simulink model "dx_hand_model"  (R2017b)
settings: Solver=ode3  StartTime=0.0  StopTime=inf  FixedStep=0.01  RelTol=1e-3  EnableMultiTasking=on
InitFcn:
  | cutFreq = 0.1; % T
  | sampleTime = 0.01;
  | filt = tf(1,[cutFreq 1]);
  | filt = c2d(filt,sampleTime);
  | 
  | cutFreq2 = 1;
  | filt2 = tf(1,[cutFreq2 1]);
  | filt2 = c2d(filt2,sampleTime);
  | 
  | cutFreq3 = 0.3;
  | filt3 = tf(1,[cutFreq3 1]);
  | filt3 = c2d(filt3,sampleTime);
  | 
  | update_param = 2;
  | 
  | ampliFactor = 1.60;
  | ampliFactorMiddle = 2.00;
  | ampliFactorDistal = 1;
  | 
  | % Set Hand Address
  | % RightHandAddress = '10.100.39.144';
  | RightHandAddress = '10.24.4.91';
  | Verosim = '10.100.39.22'
  | LeftHandAddress = '10.100.39.22'
  | 
  | max_force = 24; % Newton
model workspace (MAT data in the model file):
  SL_ROS_VariableLengthArrays_MaxSizes : struct (value not decoded)
libraries: robotlib x136, simulink_extras x27, simulink x16, etargetslib x2, dspnetwork x2
(part 15 of 19)

== matlab function dx_hand_model/Thumb/Direct Kinematics/F transformation new ==
  data: B output; C output; q_A input; F output; q_B input; F_1 output; q_C input; D output; E output; q_E input; q_J input; J output; I output
function [B,C,F,F_1, D, E, J, I]  = fcn(q_A, q_B, q_C, q_E, q_J)
T_B =[ - (4967757600021511*sin(q_A))/40564819207303340847894502572032 - (2^(1/2)*cos(q_A))/2,                                  2^(1/2)/2 - (24678615572571482867467662723121*cos(q_A))/3291009114642412084309938365114701009965471731267159726697218048 + (4967757600021511*2^(1/2)*sin(q_A))/162259276829213363391578010288128,                          (4967757600021511*cos(q_A))/40564819207303340847894502572032 + (4967757600021511*2^(1/2))/162259276829213363391578010288128 - (2^(1/2)*sin(q_A))/2,                                        (33*2^(1/2))/4;...
               (7025470172532439*cos(q_A))/81129638414606681695789005144064 - sin(q_A), - (4967757600021511*cos(q_A))/81129638414606681695789005144064 - (34900832843322459977667745295329*sin(q_A))/6582018229284824168619876730229402019930943462534319453394436096 - 7025470172532437/81129638414606681695789005144064, cos(q_A) + (7025470172532439*sin(q_A))/81129638414606681695789005144064 - 34900832843322450042152545252307/6582018229284824168619876730229402019930943462534319453394436096, -231840515693570421/162259276829213363391578010288128;...
                                                                  (2^(1/2)*cos(q_A))/2,                                                                                                                                                 2^(1/2)/2 - (4967757600021511*2^(1/2)*sin(q_A))/162259276829213363391578010288128,                                                                                         (4967757600021511*2^(1/2))/162259276829213363391578010288128 + (2^(1/2)*sin(q_A))/2,                                        (33*2^(1/2))/4;...
                                                                                     0,                                                                                                                                                                                                                                 0,                                                                                                                                                                           0,                                                     1]; 

T_C = [                    sin(q_B + pi/2)*(2^(1/2)/2 - (24678615572571482867467662723121*cos(q_A))/3291009114642412084309938365114701009965471731267159726697218048 + (4967757600021511*2^(1/2)*sin(q_A))/162259276829213363391578010288128) - cos(q_B + pi/2)*((4967757600021511*sin(q_A))/40564819207303340847894502572032 + (2^(1/2)*cos(q_A))/2),                      cos(q_B + pi/2)*(2^(1/2)/2 - (24678615572571482867467662723121*cos(q_A))/3291009114642412084309938365114701009965471731267159726697218048 + (4967757600021511*2^(1/2)*sin(q_A))/162259276829213363391578010288128) + sin(q_B + pi/2)*((4967757600021511*sin(q_A))/40564819207303340847894502572032 + (2^(1/2)*cos(q_A))/2),                          (4967757600021511*cos(q_A))/40564819207303340847894502572032 + (4967757600021511*2^(1/2))/162259276829213363391578010288128 - (2^(1/2)*sin(q_A))/2,                                                          (33*2^(1/2))/4 - 30*cos(q_B + pi/2)*((4967757600021511*sin(q_A))/40564819207303340847894502572032 + (2^(1/2)*cos(q_A))/2) + 30*sin(q_B + pi/2)*(2^(1/2)/2 - (24678615572571482867467662723121*cos(q_A))/3291009114642412084309938365114701009965471731267159726697218048 + (4967757600021511*2^(1/2)*sin(q_A))/162259276829213363391578010288128);...
 cos(q_B + pi/2)*((7025470172532439*cos(q_A))/81129638414606681695789005144064 - sin(q_A)) - sin(q_B + pi/2)*((4967757600021511*cos(q_A))/81129638414606681695789005144064 + (34900832843322459977667745295329*sin(q_A))/6582018229284824168619876730229402019930943462534319453394436096 + 7025470172532437/81129638414606681695789005144064), - cos(q_B + pi/2)*((4967757600021511*cos(q_A))/81129638414606681695789005144064 + (34900832843322459977667745295329*sin(q_A))/6582018229284824168619876730229402019930943462534319453394436096 + 7025470172532437/81129638414606681695789005144064) - sin(q_B + pi/2)*((7025470172532439*cos(q_A))/81129638414606681695789005144064 - sin(q_A)), cos(q_A) + (7025470172532439*sin(q_A))/81129638414606681695789005144064 - 34900832843322450042152545252307/6582018229284824168619876730229402019930943462534319453394436096, 30*cos(q_B + pi/2)*((7025470172532439*cos(q_A))/81129638414606681695789005144064 - sin(q_A)) - 30*sin(q_B + pi/2)*((4967757600021511*cos(q_A))/81129638414606681695789005144064 + (34900832843322459977667745295329*sin(q_A))/6582018229284824168619876730229402019930943462534319453394436096 + 7025470172532437/81129638414606681695789005144064) - 231840515693570421/162259276829213363391578010288128;...
                                                                                                                                                                                                    sin(q_B + pi/2)*(2^(1/2)/2 - (4967757600021511*2^(1/2)*sin(q_A))/162259276829213363391578010288128) + (2^(1/2)*cos(q_A)*cos(q_B + pi/2))/2,                                                                                                                                                                                                      cos(q_B + pi/2)*(2^(1/2)/2 - (4967757600021511*2^(1/2)*sin(q_A))/162259276829213363391578010288128) - (2^(1/2)*cos(q_A)*sin(q_B + pi/2))/2,                                                                                         (4967757600021511*2^(1/2))/162259276829213363391578010288128 + (2^(1/2)*sin(q_A))/2,                                                                                                                                                                                                                                              30*sin(q_B + pi/2)*(2^(1/2)/2 - (4967757600021511*2^(1/2)*sin(q_A))/162259276829213363391578010288128) + (33*2^(1/2))/4 + 15*2^(1/2)*cos(q_A)*cos(q_B + pi/2);...
                                                                                                                                                                                                                                                                                                                                 0,                                                                                                                                                                                                                                                                                                                                               0,                                                                                                                                                                           0,                                                                                                                                                                                                                                                                                                                                                                                                          1];
                                                                                                                                                                                                                                                                                                                                             
A_3 = [ cos(q_C - 2305491947385741/1125899906842624), -sin(q_C - 2305491947385741/1125899906842624), 0, 4561^(1/2)*cos(q_C - 2305491947385741/1125899906842624); ...
 sin(q_C - 2305491947385741/1125899906842624),  cos(q_C - 2305491947385741/1125899906842624), 0, 4561^(1/2)*sin(q_C - 2305491947385741/1125899906842624); ...
                                            0,                                             0, 1,                                                       0; ...
                                            0,                                             0, 0,                                                       1];
 
A_4 = [ cos(q_C - pi/2), -(4967757600021511*sin(q_C - pi/2))/81129638414606681695789005144064,                                  -sin(q_C - pi/2), 60*cos(q_C - pi/2); ...
 sin(q_C - pi/2),  (4967757600021511*cos(q_C - pi/2))/81129638414606681695789005144064,                                   cos(q_C - pi/2), 60*sin(q_C - pi/2); ...
0,                                                                   -1, 4967757600021511/81129638414606681695789005144064,                  0; ...
               0,                                                                    0,                                                 0,                  1];
 
A_D = [ cos(q_C - pi/2), -(4967757600021511*sin(q_C - pi/2))/81129638414606681695789005144064,                                  -sin(q_C - pi/2), 85*cos(q_C - pi/2); ...
 sin(q_C - pi/2),  (4967757600021511*cos(q_C - pi/2))/81129638414606681695789005144064,                                   cos(q_C - pi/2), 85*sin(q_C - pi/2); ...
               0,                                                                   -1, 4967757600021511/81129638414606681695789005144064,                  0; ...
               0,                                                                    0,                                                 0,                  1];
 
C_E = [0.0000    0.0000    1.0000   33.5857; ...
   -1.0000    0.0000    0.0000  -91.0000; ...
         0   -1.0000    0.0000    0.0000; ...
         0         0         0    1.0000];

E_J = [ cos(q_E), -(4967757600021511*sin(q_E))/81129638414606681695789005144064,                                          sin(q_E), 100*cos(q_E); ...
 sin(q_E),  (4967757600021511*cos(q_E))/81129638414606681695789005144064,                                         -cos(q_E), 100*sin(q_E); ...
        0,                                                             1, 4967757600021511/81129638414606681695789005144064,            0; ...
        0,                                                             0,                                                 0,            1];

J_I = [ 0, 0, 0,  80*sin(q_J); ...
 0, 0, 0, -80*cos(q_J); ...
 0, 0, 0,            0; ...
 0, 0, 0,            1];

T_F = T_C*A_3;
T_F_1 = T_C*A_4;
T_D = T_C*A_D;
T_E = T_C*C_E;
T_J = T_E*E_J;
T_I = T_J*J_I;

B = T_B*[ 0, 0, 0, 1]';
C = T_C*[ 0, 0, 0, 1]';
F = T_F*[ 0, 0, 0, 1]';
F_1 = T_F_1*[ 0, 0, 0, 1]';
D = T_D*[0, 0, 0, 1]';                                                                                                                                                                                                                                                                                                                                                                                                                                                                                                                                                                                                                                                                                                                                                                                         
E = T_E*[0, 0, 0, 1]';
J = T_J*[0,0,0,1]';
I = T_I*[0,0,0,1]';
end

== matlab function dx_hand_model/Thumb/Metacarphal Phalanx/MATLAB Function1 ==
  data: u input; d output
function d = fcn(u)

d = sqrt(u(1)^2+u(2)^2+u(3)^2);

== matlab function dx_hand_model/Thumb/Direct Kinematics/get H/MATLAB Function5 ==
  data: u input; d output
function d = fcn(u)

d = sqrt(u(1)^2+u(2)^2+u(3)^2);

== matlab function dx_hand_model/Thumb/Direct Kinematics/get H/MATLAB Function6 ==
  data: u input; d output
function d = fcn(u)

d = sqrt(u(1)^2+u(2)^2+u(3)^2);

== matlab function dx_hand_model/Thumb/Direct Kinematics/get H/MATLAB Function7 ==
  data: u input; d output
function d = fcn(u)

d = sqrt(u(1)^2+u(2)^2+u(3)^2);

== matlab function dx_hand_model/Thumb/Direct Kinematics/get H/MATLAB Function8 ==
  data: u input; d output
function d = fcn(u)

d = sqrt(u(1)^2+u(2)^2+u(3)^2);

== matlab function dx_hand_model/Thumb/Direct Kinematics/get H/MATLAB Function9 ==
  data: a input; xH output; b input; yH output; zH output
function [xH,yH,zH] = fcn(a,b)
if a(2) > b(2)
    xH = a(1);
    yH = a(2);
    zH = a(3);
else
    xH = b(1);
    yH = b(2);
    zH = b(3);
end

== matlab function dx_hand_model/Thumb/Direct Kinematics/get H/MATLAB Function10 ==
  data: u input; d output
function d = fcn(u)

d = sqrt(u(1)^2+u(2)^2+u(3)^2);

== matlab function dx_hand_model/Thumb/Direct Kinematics/Get G/MATLAB Function ==
  data: xI input; yI input; zI input; xH input; yH input; zH input; xD input; yD input; zD input; xG2_sol output; yG2_sol output; zG2_sol output
function [xG2_sol,yG2_sol,zG2_sol] = findG2_optimized(xI,yI,zI,xH,yH, zH, xD,yD, zD )
%function [xG2_sol,yG2_sol,zG2_sol] = findG2_optimized(xD,xH,xI,yD,yH,yI,zD,zH,zI)
%FINDG2_OPTIMIZED
%    [XG2_SOL,YG2_SOL,ZG2_SOL] = FINDG2_OPTIMIZED(XD,XH,XI,YD,YH,YI,ZD,ZH,ZI)

%    This function was generated by the Symbolic Math Toolbox version 8.0.
%    16-Feb-2018 10:54:09

t2 = xD.^2;
t3 = xH.^2;
t4 = zD.^2;
t5 = zH.^2;
t6 = yD.^2;
t7 = yI.^2;
t8 = xI.^2;
t9 = yH.^2;
t10 = zI.^2;
t11 = t4.^2;
t12 = t5.^2;
t13 = t2.*t9.*5.329e3;
t14 = t3.*t6.*5.329e3;
t15 = t2.*t7.*5.329e3;
t16 = t6.*t8.*5.329e3;
t17 = t3.*t7.*5.329e3;
t18 = t8.*t9.*5.329e3;
t19 = t2.*t5.*5.329e3;
t20 = t3.*t4.*5.329e3;
t21 = t2.*t10.*5.329e3;
t22 = t4.*t8.*5.329e3;
t23 = t3.*t10.*5.329e3;
t24 = t5.*t8.*5.329e3;
t25 = t5.*t6.*5.329e3;
t26 = t4.*t9.*5.329e3;
t27 = t6.*t10.*5.329e3;
t28 = t4.*t7.*5.329e3;
t29 = t9.*t10.*5.329e3;
t30 = t5.*t7.*5.329e3;
t31 = xD.*xH.*yD.*yI.*1.0658e4;
t32 = xD.*xI.*yD.*yH.*1.0658e4;
t33 = xD.*xH.*yH.*yI.*1.0658e4;
t34 = xH.*xI.*yD.*yH.*1.0658e4;
t35 = xD.*xI.*yH.*yI.*1.0658e4;
t36 = xH.*xI.*yD.*yI.*1.0658e4;
t37 = xD.*xH.*zD.*zI.*1.0658e4;
t38 = xD.*xI.*zD.*zH.*1.0658e4;
t39 = xD.*xH.*zH.*zI.*1.0658e4;
t40 = xH.*xI.*zD.*zH.*1.0658e4;
t41 = xD.*xI.*zH.*zI.*1.0658e4;
t42 = xH.*xI.*zD.*zI.*1.0658e4;
t43 = yD.*yH.*zD.*zI.*1.0658e4;
t44 = yD.*yI.*zD.*zH.*1.0658e4;
t45 = yD.*yH.*zH.*zI.*1.0658e4;
t46 = yH.*yI.*zD.*zH.*1.0658e4;
t47 = yD.*yI.*zH.*zI.*1.0658e4;
t48 = yH.*yI.*zD.*zI.*1.0658e4;
t74 = t7.*xD.*xH.*1.0658e4;
t75 = t9.*xD.*xI.*1.0658e4;
t76 = t6.*xH.*xI.*1.0658e4;
t77 = t10.*xD.*xH.*1.0658e4;
t78 = t5.*xD.*xI.*1.0658e4;
t79 = t4.*xH.*xI.*1.0658e4;
t80 = t2.*yH.*yI.*1.0658e4;
t81 = t3.*yD.*yI.*1.0658e4;
t82 = t8.*yD.*yH.*1.0658e4;
t83 = t10.*yD.*yH.*1.0658e4;
t84 = t5.*yD.*yI.*1.0658e4;
t85 = t4.*yH.*yI.*1.0658e4;
t86 = t2.*zH.*zI.*1.0658e4;
t87 = t3.*zD.*zI.*1.0658e4;
t88 = t8.*zD.*zH.*1.0658e4;
t89 = t6.*zH.*zI.*1.0658e4;
t90 = t9.*zD.*zI.*1.0658e4;
t91 = t7.*zD.*zH.*1.0658e4;
t92 = xD.*xH.*yD.*yH.*1.0658e4;
t93 = xD.*xI.*yD.*yI.*1.0658e4;
t94 = xH.*xI.*yH.*yI.*1.0658e4;
t95 = xD.*xH.*zD.*zH.*1.0658e4;
t96 = xD.*xI.*zD.*zI.*1.0658e4;
t97 = xH.*xI.*zH.*zI.*1.0658e4;
t98 = yD.*yH.*zD.*zH.*1.0658e4;
t99 = yD.*yI.*zD.*zI.*1.0658e4;
t100 = yH.*yI.*zH.*zI.*1.0658e4;
t49 = t13+t14+t15+t16+t17+t18+t19+t20+t21+t22+t23+t24+t25+t26+t27+t28+t29+t30+t31+t32+t33+t34+t35+t36+t37+t38+t39+t40+t41+t42+t43+t44+t45+t46+t47+t48-t74-t75-t76-t77-t78-t79-t80-t81-t82-t83-t84-t85-t86-t87-t88-t89-t90-t91-t92-t93-t94-t95-t96-t97-t98-t99-t100;
t203 = t2.*t5.*zH.*7.592e3;
t204 = t3.*t4.*zD.*3.066e3;
t205 = t4.*t8.*zD.*3.066e3;
t206 = t5.*t8.*zH.*7.592e3;
t207 = t5.*t6.*zH.*7.592e3;
t208 = t4.*t9.*zD.*3.066e3;
t209 = t4.*t7.*zD.*3.066e3;
t210 = t5.*t7.*zH.*7.592e3;
t211 = t5.*xD.*xI.*zH.*1.5184e4;
t212 = t4.*xH.*xI.*zD.*6.132e3;
t213 = t5.*yD.*yI.*zH.*1.5184e4;
t214 = t4.*yH.*yI.*zD.*6.132e3;
t215 = t2.*t9.*zD.*3.066e3;
t216 = t3.*t6.*zD.*3.066e3;
t217 = t2.*t7.*zD.*3.066e3;
t218 = t6.*t8.*zD.*3.066e3;
t219 = t2.*t9.*zH.*7.592e3;
t220 = t3.*t6.*zH.*7.592e3;
t221 = t2.*t7.*zH.*7.592e3;
t222 = t3.*t7.*zD.*3.066e3;
t223 = t6.*t8.*zH.*7.592e3;
t224 = t8.*t9.*zD.*3.066e3;
t225 = t3.*t7.*zH.*7.592e3;
t226 = t8.*t9.*zH.*7.592e3;
t227 = t2.*t5.*zD.*3.066e3;
t228 = t2.*t10.*zD.*3.066e3;
t229 = t3.*t4.*zH.*7.592e3;
t230 = t2.*t10.*zH.*7.592e3;
t231 = t2.*t5.*zI.*1.5184e4;
t232 = t3.*t10.*zD.*3.066e3;
t233 = t3.*t4.*zI.*6.132e3;
t234 = t5.*t8.*zD.*1.2118e4;
t235 = t4.*t8.*zH.*1.46e3;
t236 = t3.*t10.*zH.*7.592e3;
t237 = t5.*t6.*zD.*3.066e3;
t238 = t6.*t10.*zD.*3.066e3;
t239 = t4.*t9.*zH.*7.592e3;
t240 = t6.*t10.*zH.*7.592e3;
t241 = t5.*t6.*zI.*1.5184e4;
t242 = t9.*t10.*zD.*3.066e3;
t243 = t4.*t9.*zI.*6.132e3;
t244 = t5.*t7.*zD.*1.2118e4;
t245 = t4.*t7.*zH.*1.46e3;
t246 = t9.*t10.*zH.*7.592e3;
t247 = t7.*xD.*xH.*zD.*6.132e3;
t248 = t9.*xD.*xI.*zD.*6.132e3;
t249 = t6.*xH.*xI.*zD.*6.132e3;
t250 = t7.*xD.*xH.*zH.*1.5184e4;
t251 = t9.*xD.*xI.*zH.*1.5184e4;
t252 = t6.*xH.*xI.*zH.*1.5184e4;
t253 = t5.*xD.*xH.*zD.*1.5184e4;
t254 = t4.*xD.*xH.*zH.*6.132e3;
t255 = t10.*xD.*xH.*zD.*6.132e3;
t256 = t4.*xD.*xH.*zI.*6.132e3;
t257 = t5.*xD.*xI.*zD.*9.052e3;
t258 = t4.*xD.*xI.*zH.*6.132e3;
t259 = t2.*yH.*yI.*zD.*6.132e3;
t260 = t3.*yD.*yI.*zD.*6.132e3;
t261 = t8.*yD.*yH.*zD.*6.132e3;
t262 = t4.*xD.*xI.*zI.*6.132e3;
t263 = t10.*xD.*xH.*zH.*1.5184e4;
t264 = t5.*xD.*xH.*zI.*1.5184e4;
t265 = t5.*xH.*xI.*zD.*1.5184e4;
t266 = t4.*xH.*xI.*zH.*9.052e3;
t267 = t2.*yH.*yI.*zH.*1.5184e4;
t268 = t3.*yD.*yI.*zH.*1.5184e4;
t269 = t8.*yD.*yH.*zH.*1.5184e4;
t270 = t5.*xD.*xI.*zI.*1.5184e4;
t271 = t4.*xH.*xI.*zI.*6.132e3;
t272 = t5.*xH.*xI.*zI.*1.5184e4;
t273 = t5.*yD.*yH.*zD.*1.5184e4;
t274 = t4.*yD.*yH.*zH.*6.132e3;
t275 = t10.*yD.*yH.*zD.*6.132e3;
t276 = t4.*yD.*yH.*zI.*6.132e3;
t277 = t5.*yD.*yI.*zD.*9.052e3;
t278 = t4.*yD.*yI.*zH.*6.132e3;
t279 = t2.*zD.*zH.*zI.*6.132e3;
t280 = t4.*yD.*yI.*zI.*6.132e3;
t281 = t10.*yD.*yH.*zH.*1.5184e4;
t282 = t5.*yD.*yH.*zI.*1.5184e4;
t283 = t5.*yH.*yI.*zD.*1.5184e4;
t284 = t4.*yH.*yI.*zH.*9.052e3;
t285 = t3.*zD.*zH.*zI.*1.5184e4;
t286 = t5.*yD.*yI.*zI.*1.5184e4;
t287 = t4.*yH.*yI.*zI.*6.132e3;
t288 = t5.*yH.*yI.*zI.*1.5184e4;
t289 = t6.*zD.*zH.*zI.*6.132e3;
t290 = t9.*zD.*zH.*zI.*1.5184e4;
t291 = xD.*xH.*yD.*yH.*zD.*6.132e3;
t292 = xD.*xH.*yD.*yI.*zD.*6.132e3;
t293 = xD.*xI.*yD.*yH.*zD.*6.132e3;
t294 = xD.*xI.*yD.*yI.*zD.*6.132e3;
t295 = xD.*xH.*yD.*yH.*zH.*1.5184e4;
t296 = xD.*xH.*yD.*yI.*zH.*1.5184e4;
t297 = xD.*xH.*yH.*yI.*zD.*6.132e3;
t298 = xD.*xI.*yD.*yH.*zH.*1.5184e4;
t299 = xH.*xI.*yD.*yH.*zD.*6.132e3;
t300 = xD.*xI.*yD.*yI.*zH.*1.5184e4;
t301 = xD.*xI.*yH.*yI.*zD.*6.132e3;
t302 = xH.*xI.*yD.*yI.*zD.*6.132e3;
t303 = xD.*xH.*yH.*yI.*zH.*1.5184e4;
t304 = xH.*xI.*yD.*yH.*zH.*1.5184e4;
t305 = xD.*xI.*yH.*yI.*zH.*1.5184e4;
t306 = xH.*xI.*yD.*yI.*zH.*1.5184e4;
t307 = xH.*xI.*yH.*yI.*zD.*6.132e3;
t308 = xH.*xI.*yH.*yI.*zH.*1.5184e4;
t309 = xD.*xH.*zD.*zH.*zI.*2.1316e4;
t310 = xD.*xI.*zD.*zH.*zI.*9.052e3;
t311 = xH.*xI.*zD.*zH.*zI.*9.052e3;
t312 = yD.*yH.*zD.*zH.*zI.*2.1316e4;
t313 = yD.*yI.*zD.*zH.*zI.*9.052e3;
t314 = yH.*yI.*zD.*zH.*zI.*9.052e3;
t50 = t203+t204+t205+t206+t207+t208+t209+t210-t211-t212-t213-t214+t215+t216+t217+t218+t219+t220+t221+t222+t223+t224+t225+t226+t227+t228+t229+t230-t231+t232-t233-t234+t235+t236+t237+t238+t239+t240-t241+t242-t243-t244+t245+t246-t247-t248-t249-t250-t251-t252-t253-t254-t255+t256+t257+t258-t259-t260-t261-t262-t263+t264+t265-t266-t267-t268-t269+t270+t271-t272-t273-t274-t275+t276+t277+t278-t279-t280-t281+t282+t283-t284-t285+t286+t287-t288-t289-t290-t291+t292+t293-t294-t295+t296+t297+t298+t299-t300+t301+t302+t303+t304+t305+t306-t307-t308+t309-t310+t311+t312-t313+t314;
t51 = xD.*yH;
t52 = xI.*yD;
t53 = xH.*yI;
t56 = xH.*yD;
t57 = xD.*yI;
t58 = xI.*yH;
t54 = t51+t52+t53-t56-t57-t58;
t55 = 1.0./t54;
t59 = t3.*yD.*5.2e1;
t60 = t2.*yI.*2.1e1;
t61 = t5.*yD.*5.2e1;
t62 = t4.*yI.*2.1e1;
t63 = xD.*xH.*yD.*2.1e1;
t64 = xD.*xH.*yI.*3.1e1;
t65 = xD.*xI.*yH.*2.1e1;
t66 = xH.*xI.*yH.*5.2e1;
t67 = yD.*zD.*zH.*2.1e1;
t68 = yH.*zD.*zI.*2.1e1;
t69 = yI.*zD.*zH.*3.1e1;
t70 = yH.*zH.*zI.*5.2e1;
t71 = t59+t60+t61+t62+t63+t64+t65+t66+t67+t68+t69+t70-t2.*yH.*2.1e1-t4.*yH.*2.1e1-t3.*yI.*5.2e1-t5.*yI.*5.2e1-xD.*xI.*yD.*2.1e1-xD.*xH.*yH.*5.2e1-xH.*xI.*yD.*5.2e1-yD.*zD.*zI.*2.1e1-yH.*zD.*zH.*5.2e1-yD.*zH.*zI.*5.2e1;
t72 = zD.*(2.1e1./7.3e1);
t73 = zH.*(5.2e1./7.3e1);
t101 = 1.0./t49;
t102 = t2.*t12.*2.704e3;
t103 = t3.*t11.*4.41e2;
t104 = t8.*t11.*4.41e2;
t105 = t8.*t12.*2.704e3;
t106 = t6.*t12.*2.704e3;
t107 = t9.*t11.*4.41e2;
t108 = t7.*t11.*4.41e2;
t109 = t7.*t12.*2.704e3;
t110 = t7.*xD.*xH.*1.0913792e7;
t111 = t9.*xD.*xI.*1.0913792e7;
t112 = t6.*xH.*xI.*1.0913792e7;
t113 = t2.*yH.*yI.*1.0913792e7;
t114 = t3.*yD.*yI.*1.0913792e7;
t115 = t8.*yD.*yH.*1.0913792e7;
t116 = t2.*t5.*zD.*zH.*2.184e3;
t117 = t3.*t4.*zD.*zH.*2.184e3;
t118 = t4.*t8.*zD.*zH.*1.302e3;
t119 = t5.*t6.*zD.*zH.*2.184e3;
t120 = t4.*t9.*zD.*zH.*2.184e3;
t121 = t4.*t7.*zD.*zH.*1.302e3;
t122 = t2.*t4.*t9.*4.41e2;
t123 = t3.*t4.*t6.*4.41e2;
t124 = t2.*t4.*t7.*4.41e2;
t125 = t4.*t6.*t8.*4.41e2;
t126 = t2.*t5.*t9.*2.704e3;
t127 = t3.*t5.*t6.*2.704e3;
t128 = t2.*t5.*t7.*2.704e3;
t129 = t3.*t4.*t7.*4.41e2;
t130 = t5.*t6.*t8.*2.704e3;
t131 = t4.*t8.*t9.*4.41e2;
t132 = t3.*t5.*t7.*2.704e3;
t133 = t5.*t8.*t9.*2.704e3;
t134 = t2.*t4.*t5.*4.41e2;
t135 = t2.*t4.*t10.*4.41e2;
t136 = t3.*t4.*t5.*2.704e3;
t137 = t2.*t5.*t10.*2.704e3;
t138 = t3.*t4.*t10.*4.41e2;
t139 = t3.*t5.*t10.*2.704e3;
t140 = t4.*t5.*t6.*4.41e2;
t141 = t4.*t6.*t10.*4.41e2;
t142 = t4.*t5.*t9.*2.704e3;
t143 = t5.*t6.*t10.*2.704e3;
t144 = t4.*t9.*t10.*4.41e2;
t145 = t5.*t9.*t10.*2.704e3;
t146 = t4.*t5.*xD.*xI.*3.486e3;
t147 = t2.*t9.*zD.*zH.*2.184e3;
t148 = t3.*t6.*zD.*zH.*2.184e3;
t149 = t2.*t7.*zD.*zH.*2.184e3;
t150 = t6.*t8.*zD.*zH.*2.184e3;
t151 = t3.*t7.*zD.*zH.*2.184e3;
t152 = t8.*t9.*zD.*zH.*2.184e3;
t153 = t4.*t5.*yD.*yI.*3.486e3;
t154 = t2.*t10.*zD.*zH.*2.184e3;
t155 = t3.*t10.*zD.*zH.*2.184e3;
t156 = t6.*t10.*zD.*zH.*2.184e3;
t157 = t9.*t10.*zD.*zH.*2.184e3;
t158 = xD.*xH.*yD.*yH.*1.0913792e7;
t159 = xD.*xI.*yD.*yI.*1.0913792e7;
t160 = xH.*xI.*yH.*yI.*1.0913792e7;
t161 = t4.*xD.*xH.*zD.*zI.*8.82e2;
t162 = t5.*xD.*xI.*zD.*zH.*1.04e3;
t163 = t4.*xD.*xI.*zD.*zH.*8.82e2;
t164 = t5.*xD.*xH.*zH.*zI.*5.408e3;
t165 = t5.*xH.*xI.*zD.*zH.*5.408e3;
t166 = t5.*xD.*xI.*zH.*zI.*5.408e3;
t167 = t4.*xH.*xI.*zD.*zI.*8.82e2;
t168 = t4.*yD.*yH.*zD.*zI.*8.82e2;
t169 = t5.*yD.*yI.*zD.*zH.*1.04e3;
t170 = t4.*yD.*yI.*zD.*zH.*8.82e2;
t171 = t5.*yD.*yH.*zH.*zI.*5.408e3;
t172 = t5.*yH.*yI.*zD.*zH.*5.408e3;
t173 = t5.*yD.*yI.*zH.*zI.*5.408e3;
t174 = t4.*yH.*yI.*zD.*zI.*8.82e2;
t175 = t4.*xD.*xH.*yD.*yI.*8.82e2;
t176 = t4.*xD.*xI.*yD.*yH.*8.82e2;
t177 = t5.*xD.*xH.*yD.*yI.*5.408e3;
t178 = t4.*xD.*xH.*yH.*yI.*8.82e2;
t179 = t5.*xD.*xI.*yD.*yH.*5.408e3;
t180 = t4.*xH.*xI.*yD.*yH.*8.82e2;
t181 = t4.*xD.*xI.*yH.*yI.*8.82e2;
t182 = t4.*xH.*xI.*yD.*yI.*8.82e2;
t183 = t5.*xD.*xH.*yH.*yI.*5.408e3;
t184 = t5.*xH.*xI.*yD.*yH.*5.408e3;
t185 = t5.*xD.*xI.*yH.*yI.*5.408e3;
t186 = t5.*xH.*xI.*yD.*yI.*5.408e3;
t187 = t5.*xD.*xH.*zD.*zI.*9.776e3;
t188 = t4.*xD.*xH.*zH.*zI.*5.25e3;
t189 = t5.*xH.*xI.*zD.*zI.*1.04e3;
t190 = t4.*xH.*xI.*zH.*zI.*3.486e3;
t191 = t5.*yD.*yH.*zD.*zI.*9.776e3;
t192 = t4.*yD.*yH.*zH.*zI.*5.25e3;
t193 = t5.*yH.*yI.*zD.*zI.*1.04e3;
t194 = t4.*yH.*yI.*zH.*zI.*3.486e3;
t195 = xD.*xH.*yD.*yI.*zD.*zH.*4.368e3;
t196 = xD.*xI.*yD.*yH.*zD.*zH.*4.368e3;
t197 = xD.*xH.*yH.*yI.*zD.*zH.*4.368e3;
t198 = xH.*xI.*yD.*yH.*zD.*zH.*4.368e3;
t199 = xD.*xI.*yH.*yI.*zD.*zH.*4.368e3;
t200 = xH.*xI.*yD.*yI.*zD.*zH.*4.368e3;
t323 = t2.*t9.*5.456896e6;
t324 = t3.*t6.*5.456896e6;
t325 = t2.*t7.*5.456896e6;
t326 = t6.*t8.*5.456896e6;
t327 = t3.*t7.*5.456896e6;
t328 = t8.*t9.*5.456896e6;
t329 = t12.*xD.*xI.*5.408e3;
t330 = t11.*xH.*xI.*8.82e2;
t331 = t12.*yD.*yI.*5.408e3;
t332 = t11.*yH.*yI.*8.82e2;
t333 = t2.*t5.*zH.*zI.*5.408e3;
t334 = t3.*t4.*zD.*zI.*8.82e2;
t335 = t5.*t8.*zD.*zH.*3.224e3;
t336 = t5.*t6.*zH.*zI.*5.408e3;
t337 = t4.*t9.*zD.*zI.*8.82e2;
t338 = t5.*t7.*zD.*zH.*3.224e3;
t339 = t4.*t5.*t8.*1.223e3;
t340 = t4.*t5.*t7.*1.223e3;
t341 = t4.*t7.*xD.*xH.*8.82e2;
t342 = t4.*t9.*xD.*xI.*8.82e2;
t343 = t4.*t6.*xH.*xI.*8.82e2;
t344 = t5.*t7.*xD.*xH.*5.408e3;
t345 = t5.*t9.*xD.*xI.*5.408e3;
t346 = t5.*t6.*xH.*xI.*5.408e3;
t347 = t4.*t5.*xD.*xH.*4.368e3;
t348 = t4.*t10.*xD.*xH.*8.82e2;
t349 = t2.*t4.*yH.*yI.*8.82e2;
t350 = t3.*t4.*yD.*yI.*8.82e2;
t351 = t4.*t8.*yD.*yH.*8.82e2;
t352 = t5.*t10.*xD.*xH.*5.408e3;
t353 = t4.*t5.*xH.*xI.*1.04e3;
t354 = t2.*t5.*yH.*yI.*5.408e3;
t355 = t3.*t5.*yD.*yI.*5.408e3;
t356 = t5.*t8.*yD.*yH.*5.408e3;
t357 = t4.*t5.*yD.*yH.*4.368e3;
t358 = t4.*t10.*yD.*yH.*8.82e2;
t359 = t2.*t5.*zD.*zI.*4.368e3;
t360 = t2.*t4.*zH.*zI.*8.82e2;
t361 = t5.*t10.*yD.*yH.*5.408e3;
t362 = t4.*t5.*yH.*yI.*1.04e3;
t363 = t3.*t5.*zD.*zI.*5.408e3;
t364 = t3.*t4.*zH.*zI.*4.368e3;
t365 = t5.*t6.*zD.*zI.*4.368e3;
t366 = t4.*t6.*zH.*zI.*8.82e2;
t367 = t5.*t9.*zD.*zI.*5.408e3;
t368 = t4.*t9.*zH.*zI.*4.368e3;
t369 = xD.*xH.*yD.*yI.*1.0913792e7;
t370 = xD.*xI.*yD.*yH.*1.0913792e7;
t371 = xD.*xH.*yH.*yI.*1.0913792e7;
t372 = xH.*xI.*yD.*yH.*1.0913792e7;
t373 = xD.*xI.*yH.*yI.*1.0913792e7;
t374 = xH.*xI.*yD.*yI.*1.0913792e7;
t375 = t5.*xD.*xH.*zD.*zH.*5.408e3;
t376 = t4.*xD.*xH.*zD.*zH.*8.82e2;
t377 = t4.*xD.*xI.*zD.*zI.*8.82e2;
t378 = t4.*xH.*xI.*zD.*zH.*3.486e3;
t379 = t5.*xH.*xI.*zH.*zI.*5.408e3;
t380 = t5.*yD.*yH.*zD.*zH.*5.408e3;
t381 = t4.*yD.*yH.*zD.*zH.*8.82e2;
t382 = t4.*yD.*yI.*zD.*zI.*8.82e2;
t383 = t4.*yH.*yI.*zD.*zH.*3.486e3;
t384 = t5.*yH.*yI.*zH.*zI.*5.408e3;
t385 = t4.*xD.*xH.*yD.*yH.*8.82e2;
t386 = t4.*xD.*xI.*yD.*yI.*8.82e2;
t387 = t5.*xD.*xH.*yD.*yH.*5.408e3;
t388 = t5.*xD.*xI.*yD.*yI.*5.408e3;
t389 = t4.*xH.*xI.*yH.*yI.*8.82e2;
t390 = t5.*xH.*xI.*yH.*yI.*5.408e3;
t391 = t7.*xD.*xH.*zD.*zH.*4.368e3;
t392 = t9.*xD.*xI.*zD.*zH.*4.368e3;
t393 = t6.*xH.*xI.*zD.*zH.*4.368e3;
t394 = t10.*xD.*xH.*zD.*zH.*4.368e3;
t395 = t2.*yH.*yI.*zD.*zH.*4.368e3;
t396 = t3.*yD.*yI.*zD.*zH.*4.368e3;
t397 = t8.*yD.*yH.*zD.*zH.*4.368e3;
t398 = t5.*xD.*xI.*zD.*zI.*1.04e3;
t399 = t4.*xD.*xI.*zH.*zI.*3.486e3;
t400 = t10.*yD.*yH.*zD.*zH.*4.368e3;
t401 = t5.*yD.*yI.*zD.*zI.*1.04e3;
t402 = t4.*yD.*yI.*zH.*zI.*3.486e3;
t403 = xD.*xH.*yD.*yH.*zD.*zH.*4.368e3;
t404 = xD.*xI.*yD.*yI.*zD.*zH.*4.368e3;
t405 = xH.*xI.*yH.*yI.*zD.*zH.*4.368e3;
t201 = t102+t103+t104+t105+t106+t107+t108+t109+t110+t111+t112+t113+t114+t115+t116+t117+t118+t119+t120+t121+t122+t123+t124+t125+t126+t127+t128+t129+t130+t131+t132+t133+t134+t135+t136+t137+t138+t139+t140+t141+t142+t143+t144+t145+t146+t147+t148+t149+t150+t151+t152+t153+t154+t155+t156+t157+t158+t159+t160+t161+t162+t163+t164+t165+t166+t167+t168+t169+t170+t171+t172+t173+t174+t175+t176+t177+t178+t179+t180+t181+t182+t183+t184+t185+t186+t187+t188+t189+t190+t191+t192+t193+t194+t195+t196+t197+t198+t199+t200-t323-t324-t325-t326-t327-t328-t329-t330-t331-t332-t333-t334-t335-t336-t337-t338-t339-t340-t341-t342-t343-t344-t345-t346-t347-t348-t349-t350-t351-t352-t353-t354-t355-t356-t357-t358-t359-t360-t361-t362-t363-t364-t365-t366-t367-t368-t369-t370-t371-t372-t373-t374-t375-t376-t377-t378-t379-t380-t381-t382-t383-t384-t385-t386-t387-t388-t389-t390-t391-t392-t393-t394-t395-t396-t397-t398-t399-t400-t401-t402-t403-t404-t405;
t202 = 1.0./t49.^2;
t315 = t50.^2;
t316 = t202.*t315.*(1.0./4.0);
t406 = t101.*t201;
t317 = t316-t406;
t318 = sqrt(complex(t317));
t319 = yD.*zH;
t320 = yI.*zD;
t321 = yH.*zI;
t322 = t319+t320+t321-yH.*zD-yD.*zI-yI.*zH;
t407 = t72+t73+t318;
t408 = t9.*xD.*5.2e1;
t409 = t6.*xI.*2.1e1;
t410 = t5.*xD.*5.2e1;
t411 = t4.*xI.*2.1e1;
t412 = xD.*yD.*yH.*2.1e1;
t413 = xH.*yD.*yI.*2.1e1;
t414 = xI.*yD.*yH.*3.1e1;
t415 = xH.*yH.*yI.*5.2e1;
t416 = xD.*zD.*zH.*2.1e1;
t417 = xH.*zD.*zI.*2.1e1;
t418 = xI.*zD.*zH.*3.1e1;
t419 = xH.*zH.*zI.*5.2e1;
t420 = t408+t409+t410+t411+t412+t413+t414+t415+t416+t417+t418+t419-t4.*xH.*2.1e1-t6.*xH.*2.1e1-t5.*xI.*5.2e1-t9.*xI.*5.2e1-xD.*yD.*yI.*2.1e1-xH.*yD.*yH.*5.2e1-xD.*yH.*yI.*5.2e1-xD.*zD.*zI.*2.1e1-xH.*zD.*zH.*5.2e1-xD.*zH.*zI.*5.2e1;
t421 = t55.*t420.*(1.0./7.3e1);
t422 = t72+t73-t318;
xG2_sol = [t55.*t71.*(-1.0./7.3e1)+t55.*t322.*t407;t55.*t71.*(-1.0./7.3e1)+t55.*t322.*t422];
if nargout > 1
    t423 = xD.*zH;
    t424 = xI.*zD;
    t425 = xH.*zI;
    t426 = t423+t424+t425-xH.*zD-xD.*zI-xI.*zH;
    yG2_sol = [t421-t55.*t407.*t426;t421-t55.*t422.*t426];
end
if nargout > 2
    zG2_sol = [t407;t422];
end

== matlab function dx_hand_model/Thumb/Direct Kinematics/Get G/MATLAB Function2 ==
  data: x output; u input; y output; z output
function [x,y,z] = split(u)

x = u(1);
y = u(2);
z = u(3);

== matlab function dx_hand_model/Thumb/Direct Kinematics/Get G/MATLAB Function1 ==
  data: x output; u input; y output; z output
function [x,y,z] = split(u)

x = u(1);
y = u(2);
z = u(3);

== matlab function dx_hand_model/Thumb/Direct Kinematics/Get G/MATLAB Function4 ==
  data: u input; d output
function d = fcn(u)

d = sqrt(u(1)^2+u(2)^2+u(3)^2);

== matlab function dx_hand_model/Thumb/Direct Kinematics/Get G/MATLAB Function8 ==
  data: u input; d output
function d = fcn(u)

d = sqrt(u(1)^2+u(2)^2+u(3)^2);

== matlab function dx_hand_model/Thumb/Direct Kinematics/Get G/MATLAB Function9 ==
  data: a input; xG2 output; b input; yG2 output; zG2 output
function [xG2,yG2,zG2] = fcn(a,b)
if a(3) < b(3)
    xG2 = a(1);
    yG2 = a(2);
    zG2 = a(3);
else
    xG2 = b(1);
    yG2 = b(2);
    zG2 = b(3);
end

== matlab function dx_hand_model/Thumb/Direct Kinematics/Get G/MATLAB Function3 ==
  data: x output; u input; y output; z output
function [x,y,z] = split(u)

x = u(1);
y = u(2);
z = u(3);

== matlab function dx_hand_model/Thumb/Direct Kinematics/Get G/MATLAB Function10 ==
  data: u input; d output
function d = fcn(u)

d = sqrt(u(1)^2+u(2)^2+u(3)^2);

== matlab function dx_hand_model/Thumb/Direct Kinematics/Get G/MATLAB Function5 ==
  data: xH input; yH input; zH input; xD input; yD input; zD input; xG1 output; yG1 output; zG1 output
function [xG1,yG1,zG1] = findG1(xH,yH, zH, xD,yD, zD )
xG1 = xD + 52*(xH-xD)/73;
yG1 = yD + 52*(yH-yD)/73;
zG1 = zD + 52*(zH-zD)/73;

end

== matlab function dx_hand_model/Thumb/Direct Kinematics/Get G/MATLAB Function6 ==
  data: u input; d output
function d = fcn(u)

d = sqrt(u(1)^2+u(2)^2+u(3)^2);

== matlab function dx_hand_model/Thumb/Direct Kinematics/Get G/MATLAB Function7 ==
  data: a input; d output; b input
function d = fcn(a,b)

d = sqrt((a(1)-b(1))^2+(a(2) - b(2))^2+(a(3) - b(3))^2);

== matlab function dx_hand_model/Thumb/Proximal and Distal Phalanx/MATLAB Function1 ==
  data: x output; u input; y output; z output
function [x,y,z] = split(u)

x = u(1);
y = u(2);
z = u(3);

== matlab function dx_hand_model/Thumb/Metacarphal Phalanx/MATLAB Function ==
  data: CMC_AA input; MCP output; CMC_FE input; l_meta input; CMC input
function MCP = findMCP_pos(CMC_AA,CMC_FE,l_meta,CMC)
%FINDMCP_POS
%    MCP = FINDMCP_POS(CMC_AA,CMC_FE,L_META,XCMC,YCMC,ZCMC)

%    This function was generated by the Symbolic Math Toolbox version 8.0.
%    15-Feb-2018 11:39:36
xCMC = CMC(1);
yCMC = CMC(2);
zCMC = CMC(3);
t2 = cos(CMC_AA);
t3 = sin(CMC_FE);
t4 = cos(CMC_FE);
t5 = sin(CMC_AA);
MCP = [xCMC-l_meta.*t2.*t4+l_meta.*t3.*t5.*6.123233995736766e-17;yCMC-l_meta.*t2.*t3.*6.123233995736766e-17-l_meta.*t4.*t5;zCMC-l_meta.*t3;1.0];

== matlab function dx_hand_model/Thumb/Proximal and Distal Phalanx/MATLAB Function3 ==
  data: x output; u input; y output; z output
function [x,y,z] = split(u)

x = u(1);
y = u(2);
z = u(3);

== matlab function dx_hand_model/Ring Finger /Position-Force Architecture/Classic_Static_Problem ==
  data: Jcomponents input; y output; force_vector input
function y = fcn(Jcomponents, force_vector)
% Utilizzo la rendering strategy in the Force Space proposta da Mine
j_f = [force_vector(1);force_vector(2)];

Ja = [single(Jcomponents(1)); single(Jcomponents(3))];
% Jp = [single(Jcomponents(2)); single(Jcomponents(4))];

% J = [Ja Jp];

a_f = Ja'*j_f;

y = a_f;

== matlab function dx_hand_model/Thumb/Proximal and Distal Phalanx/MATLAB Function4 ==
  data: x output; u input; y output; z output
function [x,y,z] = split(u)

x = u(1);
y = u(2);
z = u(3);

== matlab function dx_hand_model/Thumb/Proximal and Distal Phalanx/APPROSSIMAZIONE ==
  data: MCP_FE output; CMC_FE input
function MCP_FE  = assumption(CMC_FE)

MCP_FE = pi/4-(-CMC_FE);

== matlab function dx_hand_model/Thumb/Proximal and Distal Phalanx/MATLAB Function ==
  data: CMC_AA input; xPIP_s output; CMC_FE input; MCP_AA input; MCP_FE input; l_dist input; l_meta input; xCMC input; yCMC input; zCMC input; yPIP_s output; zPIP_s output; MCP_AA_out output
function [xPIP_s,yPIP_s,zPIP_s,MCP_AA_out] = findPIP_fun(CMC_AA,CMC_FE,MCP_AA,MCP_FE,l_dist,l_meta,xCMC,yCMC,zCMC)
%FINDPIP_FUN
%    [XPIP_S,YPIP_S,ZPIP_S] = FINDPIP_FUN(CMC_AA,CMC_FE,MCP_AA,MCP_FE,L_DIST,L_META,XCMC,YCMC,ZCMC)

%    This function was generated by the Symbolic Math Toolbox version 8.0.
%    17-Feb-2018 21:06:25
[val, where] = min(abs(real(MCP_AA)));
MCP_AA = MCP_AA(where);
MCP_AA_out = MCP_AA;
t2 = sin(CMC_AA);
t3 = cos(CMC_AA);
t4 = sin(CMC_FE);
t5 = cos(CMC_FE);
t6 = cos(MCP_AA);
t7 = t2.*t4.*6.123233995736766e-17;
t8 = t7-t3.*t5;
t9 = sin(MCP_AA);
t10 = t3.*t4.*6.123233995736766e-17;
t11 = t2.*t5.*3.749399456654644e-33;
t12 = t2+t10+t11;
t13 = cos(MCP_FE);
t14 = sin(MCP_FE);
xPIP_s = xCMC+l_dist.*t13.*(t6.*t8+t9.*t12)+l_dist.*t14.*(t2.*(-6.123233995736766e-17)+t2.*t5.*6.123233995736766e-17+t3.*t4-t8.*t9.*6.123233995736766e-17+t6.*t12.*6.123233995736766e-17)+l_meta.*t2.*t4.*6.123233995736766e-17-l_meta.*t3.*t5;
if nargout > 1
    t15 = t2.*t5;
    t16 = t10+t15;
    t17 = t3.*t5.*3.749399456654644e-33;
    t18 = t3-t7+t17;
    yPIP_s = yCMC-l_dist.*t13.*(t6.*t16+t9.*t18)+l_dist.*t14.*(t3.*6.123233995736766e-17+t2.*t4-t3.*t5.*6.123233995736766e-17-t6.*t18.*6.123233995736766e-17+t9.*t16.*6.123233995736766e-17)-l_meta.*t2.*t5-l_meta.*t3.*t4.*6.123233995736766e-17;
end
if nargout > 2
    t19 = t5.*6.123233995736766e-17;
    t20 = t19-6.123233995736766e-17;
    zPIP_s = zCMC-l_meta.*t4-l_dist.*t13.*(t4.*t6+t9.*t20)-l_dist.*t14.*(t5-t4.*t9.*6.123233995736766e-17+t6.*t20.*6.123233995736766e-17+3.749399456654644e-33);
end

== matlab function dx_hand_model/Thumb/Proximal and Distal Phalanx/MATLAB Function5 ==
  data: x output; u input; y output; z output
function [x,y,z] = split(u)

x = u(1);
y = u(2);
z = u(3);
